simulink library "RRProbotLibrary"  (R2020b)
settings: Solver=VariableStepAuto  StartTime=0.0  StopTime=10.0  RelTol=1e-3
undefined symbols (not defined in the file): DiscIntNeverNeededParam, elbows, H, K, L, M, P0, Pf, T
libraries: $bdroot x7
settings Model: Creator=alons  LastModifiedBy=alons

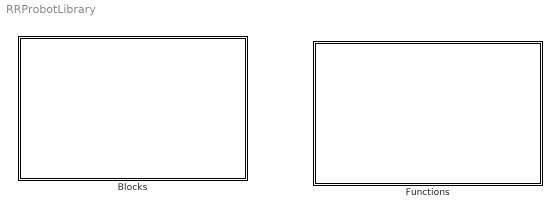
== system RRProbotLibrary ==
  Blocks : Subsystem
  Functions : Subsystem

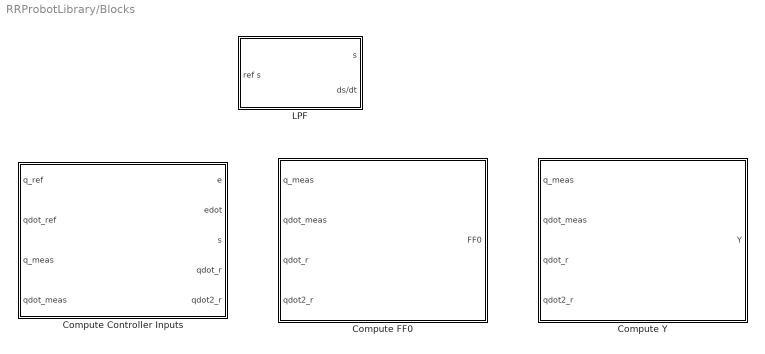
== system RRProbotLibrary/Blocks ==
  Compute Controller Inputs : Subsystem  TreatAsAtomicUnit=on  mask{K=K, LPF_f=0, LPF_s0=0}
  Compute FF0 : Subsystem  TreatAsAtomicUnit=on
  Compute Y : Subsystem  TreatAsAtomicUnit=on
  LPF : Subsystem  mask{Freq=10, s0=0}
      mask prompts: Freq "LPF Freq [Hz]"
      mask Display: fprintf('LPF %g[Hz]',Freq);

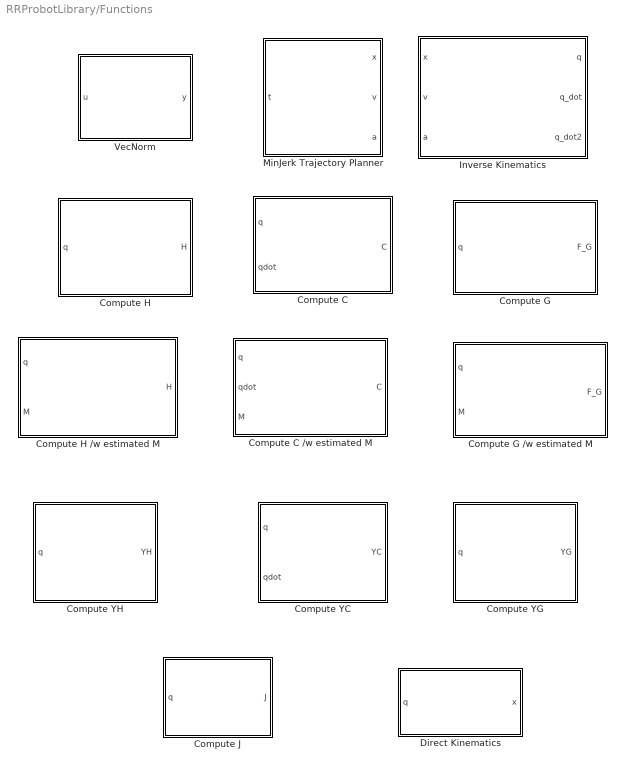
== system RRProbotLibrary/Functions ==
  Compute C : Subsystem  mask{M=M}
      mask prompts: M "M [kg]"
      mask Display: disp('Compute C')
  Compute C /w estimated M : Subsystem
      mask Display: fprintf('Compute C\n/w estimated M')
  Compute G : Subsystem  mask{M=M}
      mask prompts: M "M [kg]"
      mask Display: disp('Compute G');
  Compute G /w estimated M : Subsystem
      mask Display: fprintf('Compute G\n/w estimated M');
  Compute H : Subsystem  mask{M=M}
      mask prompts: M "M [kg]"
      mask Display: disp('Compute H');
  Compute H /w estimated M : Subsystem
      mask Display: fprintf('Compute H\n/w estimated M');
  Compute J : Subsystem
      mask Display: disp('Compute J');
  Compute YC : Subsystem
      mask Display: disp('Compute YC');
  Compute YG : Subsystem
      mask Display: disp('Compute YG');
  Compute YH : Subsystem
      mask Display: disp('Compute YH')
  Direct Kinematics : Subsystem
      mask Display: disp('Direct Kinematics');
  Inverse Kinematics : Subsystem  mask{elbows=elbows, H=H, L=L}
      mask prompts: elbows "elbows [+-1,+-1]"; H "H [m]"; L "L [m]"
      mask Display: disp('Inverse Kinematics')
  MinJerk Trajectory Planner : Subsystem  mask{P0=P0, Pf=Pf, T=T}
      mask prompts: P0 "P0 [x;y;z]"; Pf "Pf [x;y;z]"; T "T [s]"
      mask Display: fprintf('MinJerk\nTrajectory Planner')
  VecNorm : Subsystem
      mask Display: disp('VecNorm')

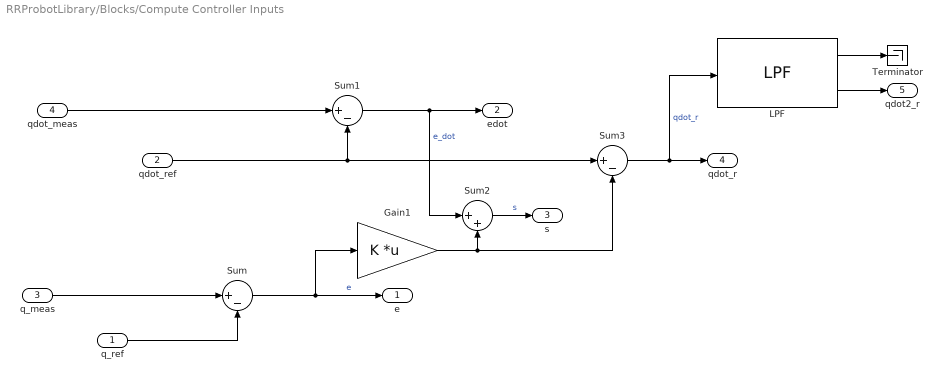
== system RRProbotLibrary/Blocks/Compute Controller Inputs ==
  q_ref : Inport  PortDimensions=3
  qdot_ref : Inport  Port=2  PortDimensions=3
  q_meas : Inport  Port=3  PortDimensions=3
  qdot_meas : Inport  Port=4  PortDimensions=3
  Gain1 : Gain  Gain=K  Multiplication=Matrix(K*u)
  LPF : $bdroot/Blocks/LPF  Freq=10  s0=0
  Sum : Sum  Inputs=|+-
  Sum1 : Sum  Inputs=|+-
  Sum2 : Sum  Inputs=|++
  Sum3 : Sum  Inputs=|+-
  Terminator : Terminator
  e : Outport
  edot : Outport  Port=2
  s : Outport  Port=3
  qdot_r : Outport  Port=4
  qdot2_r : Outport  Port=5
  wires:
  qdot_meas/1 -> Sum1/1
  Sum1/1 -> edot/1, Sum2/1  "e_dot"
  Gain1/1 -> Sum3/2, Sum2/2
  q_meas/1 -> Sum/1
  qdot_ref/1 -> Sum1/2, Sum3/1
  q_ref/1 -> Sum/2
  Sum/1 -> e/1, Gain1/1  "e"
  Sum2/1 -> s/1  "s"
  Sum3/1 -> LPF/1, qdot_r/1  "qdot_r"
  LPF/2 -> qdot2_r/1
  LPF/1 -> Terminator/1

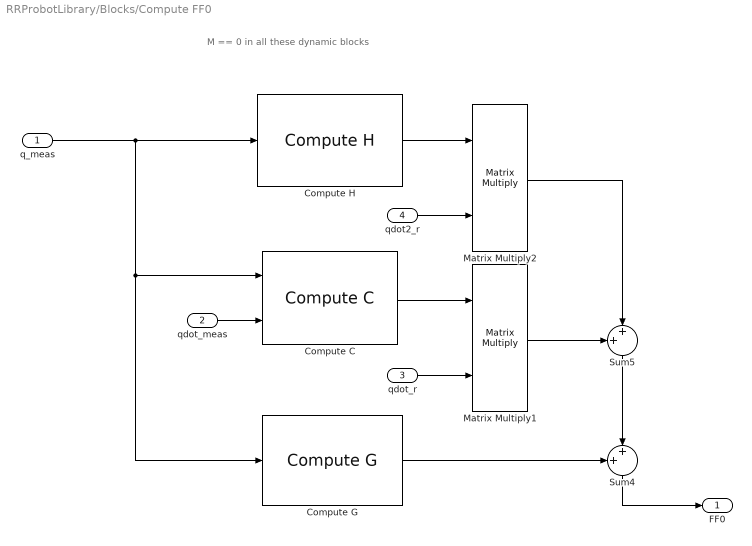
== system RRProbotLibrary/Blocks/Compute FF0 ==
  note: M == 0 in all these dynamic blocks
  q_meas : Inport
  qdot_meas : Inport  Port=2
  qdot_r : Inport  Port=3
  qdot2_r : Inport  Port=4
  Compute C : $bdroot/Functions/Compute C  M=0
  Compute G : $bdroot/Functions/Compute G  M=0
  Compute H : $bdroot/Functions/Compute H  M=0
  Matrix Multiply1 : Product  Multiplication=Matrix(*)
  Matrix Multiply2 : Product  Multiplication=Matrix(*)
  Sum4 : Sum  Inputs=++|
  Sum5 : Sum  Inputs=++|
  FF0 : Outport
  wires:
  q_meas/1 -> Compute H/1, Compute C/1, Compute G/1
  qdot_meas/1 -> Compute C/2
  Compute H/1 -> Matrix Multiply2/1
  Compute C/1 -> Matrix Multiply1/1
  Sum5/1 -> Sum4/2
  Matrix Multiply1/1 -> Sum5/1
  Matrix Multiply2/1 -> Sum5/2
  Compute G/1 -> Sum4/1
  Sum4/1 -> FF0/1
  qdot_r/1 -> Matrix Multiply1/2
  qdot2_r/1 -> Matrix Multiply2/2

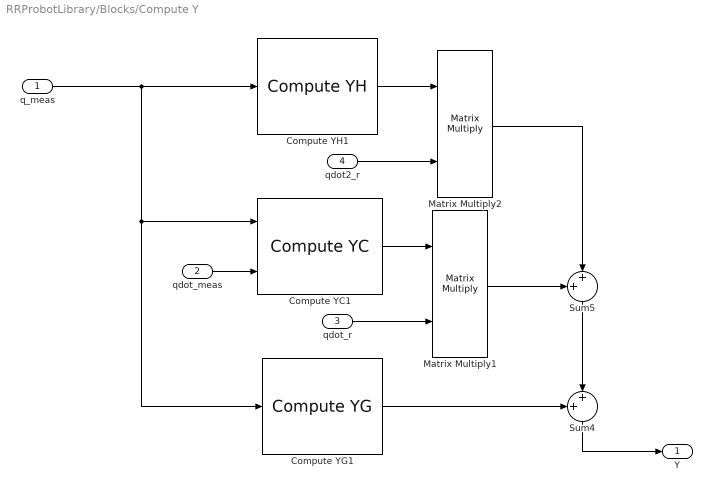
== system RRProbotLibrary/Blocks/Compute Y ==
  q_meas : Inport
  qdot_meas : Inport  Port=2
  qdot_r : Inport  Port=3
  qdot2_r : Inport  Port=4
  Compute YC1 : $bdroot/Functions/Compute YC  SystemSampleTime=-1  VariantActivationTime=update diagram  Latency=0  AutoFrameSizeCalculation=off
  Compute YG1 : $bdroot/Functions/Compute YG  SystemSampleTime=-1  VariantActivationTime=update diagram  Latency=0  AutoFrameSizeCalculation=off
  Compute YH1 : $bdroot/Functions/Compute YH  SystemSampleTime=-1  VariantActivationTime=update diagram  Latency=0  AutoFrameSizeCalculation=off
  Matrix Multiply1 : Product  Multiplication=Matrix(*)
  Matrix Multiply2 : Product  Multiplication=Matrix(*)
  Sum4 : Sum  Inputs=++|
  Sum5 : Sum  Inputs=++|
  Y : Outport
  wires:
  q_meas/1 -> Compute YH1/1, Compute YG1/1, Compute YC1/1
  qdot_meas/1 -> Compute YC1/2
  Compute YH1/1 -> Matrix Multiply2/1
  Compute YC1/1 -> Matrix Multiply1/1
  Sum5/1 -> Sum4/2
  Matrix Multiply1/1 -> Sum5/1
  Matrix Multiply2/1 -> Sum5/2
  Compute YG1/1 -> Sum4/1
  Sum4/1 -> Y/1
  qdot_r/1 -> Matrix Multiply1/2
  qdot2_r/1 -> Matrix Multiply2/2

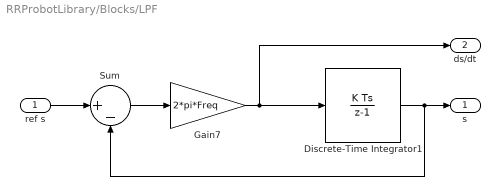
== system RRProbotLibrary/Blocks/LPF ==
  ref s : Inport
  Discrete-Time Integrator1 : DiscreteIntegrator  InitialCondition=s0  SampleTime=-1  ICPrevOutput=DiscIntNeverNeededParam  ICPrevScaledInput=DiscIntNeverNeededParam
  Gain7 : Gain  Gain=2*pi*Freq
  Sum : Sum  Inputs=|+-
  s : Outport  VectorParamsAs1DForOutWhenUnconnected=off
  ds/dt : Outport  Port=2  VectorParamsAs1DForOutWhenUnconnected=off
  wires:
  Discrete-Time Integrator1/1 -> Sum/2, s/1
  Sum/1 -> Gain7/1
  ref s/1 -> Sum/1
  Gain7/1 -> ds/dt/1, Discrete-Time Integrator1/1

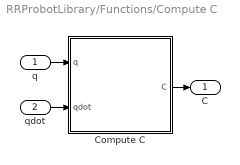
== system RRProbotLibrary/Functions/Compute C ==
  q : Inport
  qdot : Inport  Port=2
  Compute C : MATLAB Function  TreatAsAtomicUnit=on  mask{M=M}
      mask prompts: M "M [kg]"
  C : Outport
  wires:
  qdot/1 -> Compute C/2(qdot)
  q/1 -> Compute C/1(q)
  Compute C/1(C) -> C/1

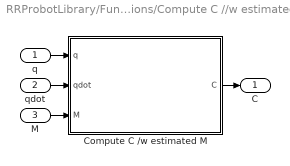
== system RRProbotLibrary/Functions/Compute C //w estimated M ==
  q : Inport
  qdot : Inport  Port=2
  M : Inport  Port=3
  Compute C /w estimated M : MATLAB Function  TreatAsAtomicUnit=on
  C : Outport
  wires:
  qdot/1 -> Compute C /w estimated M/2(qdot)
  M/1 -> Compute C /w estimated M/3(M)
  q/1 -> Compute C /w estimated M/1(q)
  Compute C /w estimated M/1(C) -> C/1

== system RRProbotLibrary/Functions/Compute G ==
  q : Inport
  Compute G : MATLAB Function  TreatAsAtomicUnit=on  mask{M=M}
      mask prompts: M "M [kg]"
  F_G : Outport
  wires:
  q/1 -> Compute G/1(q)
  Compute G/1(G) -> F_G/1  "F_G"

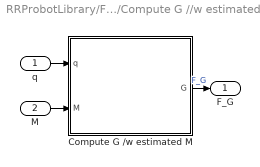
== system RRProbotLibrary/Functions/Compute G //w estimated M ==
  q : Inport
  M : Inport  Port=2
  Compute G /w estimated M : MATLAB Function  TreatAsAtomicUnit=on
  F_G : Outport
  wires:
  q/1 -> Compute G /w estimated M/1(q)
  Compute G /w estimated M/1(G) -> F_G/1  "F_G"
  M/1 -> Compute G /w estimated M/2(M)

== system RRProbotLibrary/Functions/Compute H ==
  q : Inport
  Compute H : MATLAB Function  TreatAsAtomicUnit=on  mask{M=M}
      mask prompts: M "M [kg]"
  H : Outport
  wires:
  Compute H/1(H) -> H/1
  q/1 -> Compute H/1(q)

== system RRProbotLibrary/Functions/Compute H //w estimated M ==
  q : Inport
  M : Inport  Port=2
  Compute H /w estimated M : MATLAB Function  TreatAsAtomicUnit=on
  H : Outport
  wires:
  Compute H /w estimated M/1(H) -> H/1
  q/1 -> Compute H /w estimated M/1(q)
  M/1 -> Compute H /w estimated M/2(M)

== system RRProbotLibrary/Functions/Compute J ==
  q : Inport
  Compute J : MATLAB Function  TreatAsAtomicUnit=on
  J : Outport
  wires:
  q/1 -> Compute J/1(q)
  Compute J/1(J) -> J/1

== system RRProbotLibrary/Functions/Compute YC ==
  q : Inport
  qdot : Inport  Port=2
  Compute YC : MATLAB Function  TreatAsAtomicUnit=on
  YC : Outport
  wires:
  Compute YC/1(YC) -> YC/1
  qdot/1 -> Compute YC/2(qdot)
  q/1 -> Compute YC/1(q)

== system RRProbotLibrary/Functions/Compute YG ==
  q : Inport
  Compute YG : MATLAB Function  TreatAsAtomicUnit=on
  YG : Outport
  wires:
  q/1 -> Compute YG/1(q)
  Compute YG/1(YG) -> YG/1

== system RRProbotLibrary/Functions/Compute YH ==
  q : Inport
  Compute YH : MATLAB Function  TreatAsAtomicUnit=on
  YH : Outport
  wires:
  Compute YH/1(YH) -> YH/1
  q/1 -> Compute YH/1(q)

== system RRProbotLibrary/Functions/Direct Kinematics ==
  q : Inport
  Direct Kinematics : MATLAB Function  TreatAsAtomicUnit=on
  x : Outport
  wires:
  q/1 -> Direct Kinematics/1(q)
  Direct Kinematics/1(x) -> x/1

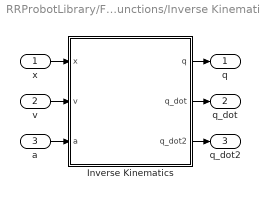
== system RRProbotLibrary/Functions/Inverse Kinematics ==
  x : Inport
  v : Inport  Port=2
  a : Inport  Port=3
  Inverse Kinematics : MATLAB Function  TreatAsAtomicUnit=on  mask{elbows=elbows, H=H, L=L}
      mask prompts: elbows "elbows [+-1,+-1]"; H "H [m]"; L "L [m]"
  q : Outport
  q_dot : Outport  Port=2
  q_dot2 : Outport  Port=3
  wires:
  a/1 -> Inverse Kinematics/3(a)
  x/1 -> Inverse Kinematics/1(x)
  Inverse Kinematics/2(q_dot) -> q_dot/1
  Inverse Kinematics/1(q) -> q/1
  v/1 -> Inverse Kinematics/2(v)
  Inverse Kinematics/3(q_dot2) -> q_dot2/1

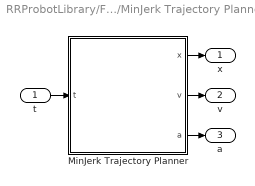
== system RRProbotLibrary/Functions/MinJerk Trajectory Planner ==
  t : Inport
  MinJerk Trajectory Planner : MATLAB Function  TreatAsAtomicUnit=on  mask{P0=P0, Pf=Pf, T=T}
      mask prompts: P0 "P0 [x;y;z]"; Pf "Pf [x;y;z]"; T "T [s]"
  x : Outport
  v : Outport  Port=2
  a : Outport  Port=3
  wires:
  MinJerk Trajectory Planner/2(v) -> v/1
  MinJerk Trajectory Planner/1(x) -> x/1
  MinJerk Trajectory Planner/3(a) -> a/1
  t/1 -> MinJerk Trajectory Planner/1(t)

== system RRProbotLibrary/Functions/VecNorm ==
  u : Inport
  VecNorm : MATLAB Function  TreatAsAtomicUnit=on
  y : Outport
  wires:
  u/1 -> VecNorm/1(u)
  VecNorm/1(y) -> y/1

== matlab function RRProbotLibrary/Functions/Compute C/Compute C ==
  data: q input size=3; C output size=[3,3]; qdot input size=3; M parameter size=1
function C = ComputeC(q,qdot,M)
C=f_Cdyn(q,qdot,M);
end

== matlab function RRProbotLibrary/Functions/Compute G/Compute G ==
  data: q input size=3; G output size=3; M parameter size=1
function G = ComputeG(q,M)
G=f_Gdyn(q,M);
end

== matlab function RRProbotLibrary/Functions/Compute H/Compute H ==
  data: q input double size=3; H output double size=[3,3]; M parameter double size=1
function H = ComputeH(q,M)
H=f_Hdyn(q,M);
end

== matlab function RRProbotLibrary/Functions/VecNorm/VecNorm ==
  data: u input; y output
function y = vecNorm2(u)
y=vecnorm(u,2);

== matlab function RRProbotLibrary/Functions/Compute C //w estimated M/Compute C //w estimated M ==
  data: q input size=3; C output size=[3,3]; qdot input size=3; M input size=1
function C = ComputeC_EstimatedM(q,qdot,M)
C=f_Cdyn(q,qdot,M);
end

== matlab function RRProbotLibrary/Functions/Compute J/Compute J ==
  data: q input size=3; J output size=[6,3]
function J = ComputeJ(q)
JL=f_JL(q);
JA=f_JA(q);
J=[JL;JA];
end

== matlab function RRProbotLibrary/Functions/Compute G //w estimated M/Compute G //w estimated M ==
  data: q input size=3; G output size=3; M input size=1
function G = ComputeG_EstimatedM(q,M)
G=f_Gdyn(q,M);
end

== matlab function RRProbotLibrary/Functions/Compute H //w estimated M/Compute H //w estimated M ==
  data: q input double size=3; H output double size=[3,3]; M input double size=1
function H = ComputeH_EstimatedM(q,M)
H=f_Hdyn(q,M);
end

== matlab function RRProbotLibrary/Functions/Compute YH/Compute YH ==
  data: q input double size=3; YH output double size=[3,3]
function YH = ComputeYH(q)
YH=f_YH(q);
end

== matlab function RRProbotLibrary/Functions/Direct Kinematics/Direct Kinematics ==
  data: x output size=3; q input size=3
function x = DirectKinematics(q)
f_A3t0=@(in1)reshape([cos(in1(1,:)),sin(in1(1,:)),0.0,0.0,-cos(in1(2,:)).*sin(in1(1,:)),cos(in1(1,:)).*cos(in1(2,:)),sin(in1(2,:)),0.0,sin(in1(1,:)).*sin(in1(2,:)),-cos(in1(1,:)).*sin(in1(2,:)),cos(in1(2,:)),0.0,cos(in1(1,:))./1.0e+1+in1(3,:).*sin(in1(1,:)).*sin(in1(2,:)),sin(in1(1,:))./1.0e+1-in1(3,:).*cos(in1(1,:)).*sin(in1(2,:)),in1(3,:).*cos(in1(2,:))+1.0./5.0,1.0],[4,4]);
A=f_A3t0(q);
x=A(1:3,4);
end

== matlab function RRProbotLibrary/Functions/Compute YC/Compute YC ==
  data: q input double size=3; YC output double size=[3,3]; qdot input
function YC = ComputeYH(q,qdot)
YC=f_YC(q,qdot);
end

== matlab function RRProbotLibrary/Functions/Compute YG/Compute YG ==
  data: q input double size=3; YG output double size=[3,1]
function YG = ComputeYG(q)
YG=f_YG(q);
end

== matlab function RRProbotLibrary/Functions/MinJerk Trajectory Planner/MinJerk Trajectory Planner ==
  data: t input; x output; v output; a output; P0 parameter size=3; Pf parameter size=3; T parameter size=1
function [x,v,a] = t2xyz(t,P0,Pf,T)
if t<T
    dP=Pf-P0;
    x=(10*(t/T)^3-15*(t/T)^4+6*(t/T)^5)*dP+P0;
    v=(30*(t^2)/T^3-60*(t^3)/T^4+30*(t^4)/T^5)*dP;
    a=(60*t/T^3-180*(t^2)/T^4+120*(t^3)/T^5)*dP;
else
    x=Pf;
    v=zeros(3,1);
    a=zeros(3,1);
end

== matlab function RRProbotLibrary/Functions/Inverse Kinematics/Inverse Kinematics ==
  data: x input size=3; v input size=3; a input size=3; q output size=3; q_dot output size=3; q_dot2 output size=3; elbows parameter size=2; H parameter size=1; L parameter size=1
function [q,q_dot,q_dot2] = xyz2q(x,v,a,elbows,H,L)
q=inverse_kin(x,H,L,elbows);

JL=f_JL(q);
q_dot=linsolve((JL),v);

JL_dot=f_JLdot(q,q_dot);
q_dot2=linsolve(JL,a-JL_dot*q_dot);
end

function q=inverse_kin(x,H,L,elbows)
t2_elbow=elbows(1);
d3_elbow=elbows(2);
q=zeros(3,size(x,2));
for i=1:size(x,2)
    %Parse
    Px=x(1,i);
    Py=x(2,i);
    Pz=x(3,i);
    %Compute d3
    d3=d3_elbow*sqrt(Px^2+Py^2+(Pz-H)^2-L^2);
    %compute theta2
    c2=(Pz-H)/(d3+eps); %<------------Added eps
    s2=t2_elbow*sqrt(1-c2^2);
    t2=atan2(s2,c2);
    %compute theta1
    a=d3*s2;
    b=L;
    c=-Py;
    d=Px;
    t1=atan2(a*d-b*c,a*c+b*d);
    %create joint vector
    q(:,i)=[t1,t2,d3]';
end
end
